simulink model "mSFunction_DaolibaiLianxi"  (Simulink 9.1)
settings: Solver=VariableStepAuto  StartTime=0.0  StopTime=10.0  RelTol=1e-3
PreLoadFcn:
  | K1=0.994475318464968;
  | K2=2.365734779560844;
  | K3=40.772814639268900;
  | K4=10.736019334899419;
libraries: checkpacklib x2
settings Model: Creator=McQueen_Zero  LastModifiedBy=McQueen_Zero
settings DataIOCC: SaveFormat=Dataset
settings OptimizationCC: LifeSpan=auto
settings DebuggingCC: UnderspecifiedInitializationDetection=Simplified  MergeDetectMultiDrivingBlocksExec=error  SFUnexpectedBacktrackingDiag=error  SFNoUnconditionalDefaultTransitionDiag=error  SFExecutionAtInitializationDiag=warning
settings HardwareCC: ProdBitPerPointer=64  ProdBitPerSizeT=64  ProdBitPerPtrDiffT=64  ProdLargestAtomicFloat=Float  ProdIntDivRoundTo=Zero  ProdEndianess=LittleEndian  ProdWordSize=64  ProdHWDeviceType=Intel->x86-64 (Windows64)
settings ModelReferenceCC: PropagateSignalLabelsOutOfModel=on
settings CodeAppCC: StateflowObjectComments=off
settings GRTTargetCC: TargetLangStandard=C99 (ISO)  CombineOutputUpdateFcns=on  GRTInterface=off
settings ConfigComp: CovMetricSettings=dwe  CovHtmlReporting=off  CovSaveCumulativeToWorkspaceVar=off  CovSaveSingleToWorkspaceVar=off  CovExternalEMLEnable=on

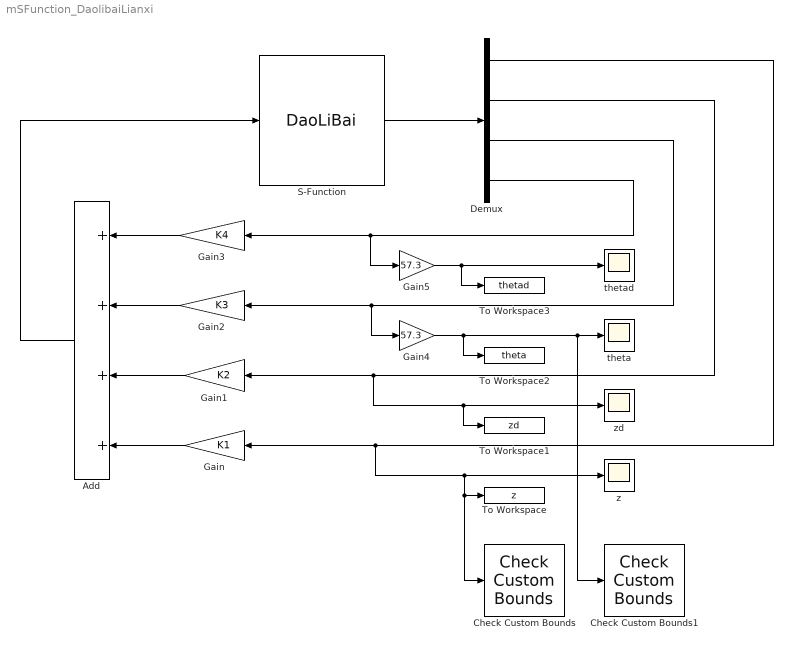
== system mSFunction_DaolibaiLianxi ==
  Add : Sum  Inputs=4
  Check Custom Bounds : checkpacklib/Check Custom Bounds  InstantiateOnLoad=on  enabled=on  stopWhenAssertionFail=off  export=off  ViewDlgPos=[]  OpenViewOnLoad=off  LaunchViewOnOpen=off  TimeUnits=seconds  EnableUpperBound=on  UpperBoundTimes=[8 10]  UpperBoundAmplitudes=[0.01 0.01];  EnableLowerBound=on  LowerBoundTimes=[8 10]  LowerBoundAmplitudes=[-0.01 -0.01]
  Check Custom Bounds1 : checkpacklib/Check Custom Bounds  InstantiateOnLoad=on  enabled=on  stopWhenAssertionFail=off  export=off  ViewDlgPos=[]  OpenViewOnLoad=off  LaunchViewOnOpen=off  TimeUnits=seconds  EnableUpperBound=on  UpperBoundTimes=[8 10]  UpperBoundAmplitudes=[0.01 0.01];  EnableLowerBound=on  LowerBoundTimes=[8 10]  LowerBoundAmplitudes=[-0.01 -0.01]
  Demux : Demux
  Gain : Gain  Gain=K1
  Gain1 : Gain  Gain=K2
  Gain2 : Gain  Gain=K3
  Gain3 : Gain  Gain=K4
  Gain4 : Gain  Gain=57.3
  Gain5 : Gain  Gain=57.3
  S-Function : S-Function  FunctionName=DaoLiBai  Parameters=1,0.2,2  SFunctionDeploymentMode=off  EnableBusSupport=off
  To Workspace : ToWorkspace  VariableName=z  SaveFormat=Timeseries  SampleTime=-1
  To Workspace1 : ToWorkspace  VariableName=zd  SaveFormat=Timeseries  SampleTime=-1
  To Workspace2 : ToWorkspace  VariableName=theta  SaveFormat=Timeseries  SampleTime=-1
  To Workspace3 : ToWorkspace  VariableName=thetad  SaveFormat=Timeseries  SampleTime=-1
  theta : Scope
  thetad : Scope
  z : Scope
  zd : Scope
  wires:
  Add/1 -> S-Function/1
  S-Function/1 -> Demux/1
  Demux/1 -> Check Custom Bounds/1, To Workspace/1, z/1, Gain/1
  Demux/2 -> To Workspace1/1, zd/1, Gain1/1
  Demux/3 -> Gain4/1, Gain2/1
  Gain/1 -> Add/4
  Gain1/1 -> Add/3
  Gain2/1 -> Add/2
  Gain3/1 -> Add/1
  Demux/4 -> Gain5/1, Gain3/1
  Gain4/1 -> To Workspace2/1, Check Custom Bounds1/1, theta/1
  Gain5/1 -> To Workspace3/1, thetad/1
